simulink model "spring_mass_model_01"  (R2014a)
settings: Solver=FixedStepDiscrete  StartTime=0.0  StopTime=inf  FixedStep=sample_time  RelTol=1e-3
values from neighbouring files (symbols this model uses):
  sample_time = 1/update_freq    (= 0.001)    [init_spring_mass_model_01.m]
undefined symbols (not defined in the file or in its folder): boom_mount_angle, c_energy, contact_threshold, control_start_time, d_y_boom_com_offset, d_y_boom_hip_offset, d_y_mount_to_com, desired_torso_angle, DiscIntNeverNeededParam, dt_thrust, dx_avg_desired, extra_leg_damping, F_thrust, fcut_contact, ff_energy_l, ff_energy_r, g, g_reduced, h_boom, i_limit_lateral, initial_com_height, initial_dt, initial_dx, j_leg, k0_virtual, k_placement, k_sea, kd_flight, kd_lateral, kd_leg_angle, kd_leg_length_secondary, kd_torso, kd_virtual, ki_lateral, kp_flight_max, kp_flight_min, kp_lateral, kp_leg_angle, kp_leg_length_secondary, kp_torso, kp_virtual, l0_virtual, l_boom, l_boom_projected, l_max, l_min, l_retract, l_seg, lambda1, lambda2, lateral_offset, LEG_MTR_MAX_TORQUE, loaded_threshold, m_leg_motor, m_total_real, max_k_virtual, max_leg_angle, max_torque_lateral, min_k_virtual, min_leg_angle ... (+6)
libraries: simulink x22
(part 1 of 2)
settings Model: xpc_rtwmakecfg_data=_xpcethercatlib_  BufferReuse=off  Creator=wmartin  LastModifiedBy=wmartin
settings SolverCC: EnableConcurrentExecution=on
settings DataIOCC: MaxDataPoints=1000000000  SaveFormat=StructureWithTime
settings OptimizationCC: BlockReduction=off  OptimizeBlockIOStorage=off  BufferReuse=off  GlobalBufferReuse=off  ExpressionFolding=off  ExpressionDepthLimit=2147483647  LocalBlockOutputs=off
settings DebuggingCC: UnderspecifiedInitializationDetection=Classic  StateNameClashWarn=warning
settings HardwareCC: ProdIntDivRoundTo=Zero  ProdEndianess=LittleEndian  ProdHWDeviceType=Generic->32-bit x86 compatible
settings RTWCC: SystemTargetFile=slrt.tlc  TemplateMakefile=slrt_default_tmf  Description=Simulink Real-Time  RTWVerbose=off  ProcessScript=slrt_make_rtw_hook  RTWCompilerOptimization=On
settings SimulinkRealTimeCC: GeneratePreprocessorConditionals=Disable all  EnableShiftOperators=on  RL32LogBufSizeModifier=100000000

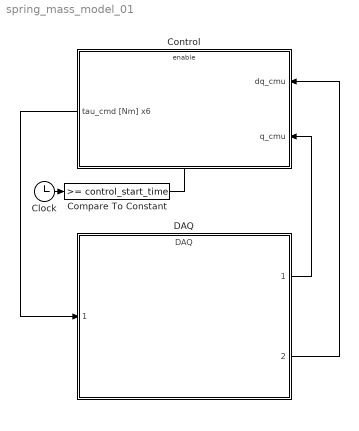
== system spring_mass_model_01 ==
  Clock : Clock
  Compare To Constant : simulink/Logic and Bit Operations/Compare To Constant  relop=>=  const=control_start_time  OutDataTypeStr=boolean
  Control : Subsystem
  DAQ : ModelReference  ModelNameDialog=DAQ  SimulationMode=Normal  ModelReferenceVersion=1.1410  CopyOfModelName=DAQ  DefaultDataLogging=on
  wires:
  DAQ/1 -> Control/2(q_cmu)
  DAQ/2 -> Control/1(dq_cmu)
  Clock/1 -> Compare To Constant/1
  Compare To Constant/1 -> Control/Enable
  Control/1(tau_cmd [Nm] x6) -> DAQ/1

== system spring_mass_model_01/Control ==
  dq_cmu : Inport
  q_cmu : Inport  Port=2
  Enable : EnablePort  StatesWhenEnabling=reset
  Actuator Control : ModelReference  ModelNameDialog=Actuator_Control  SimulationMode=Normal  ModelReferenceVersion=1.5  CopyOfModelName=Actuator_Control  DefaultDataLogging=on
  Behavior Control : Subsystem
  tau_cmd [Nm] x6 : Outport  InitialOutput=[0 0 0 0 0 0]
  wires:
  Behavior Control/1(motor_torque_cmd) -> Actuator Control/1
  dq_cmu/1 -> Actuator Control/3, Behavior Control/1(dq_cmu)
  Actuator Control/1 -> tau_cmd [Nm] x6/1
  q_cmu/1 -> Actuator Control/2, Behavior Control/2(q_cmu)

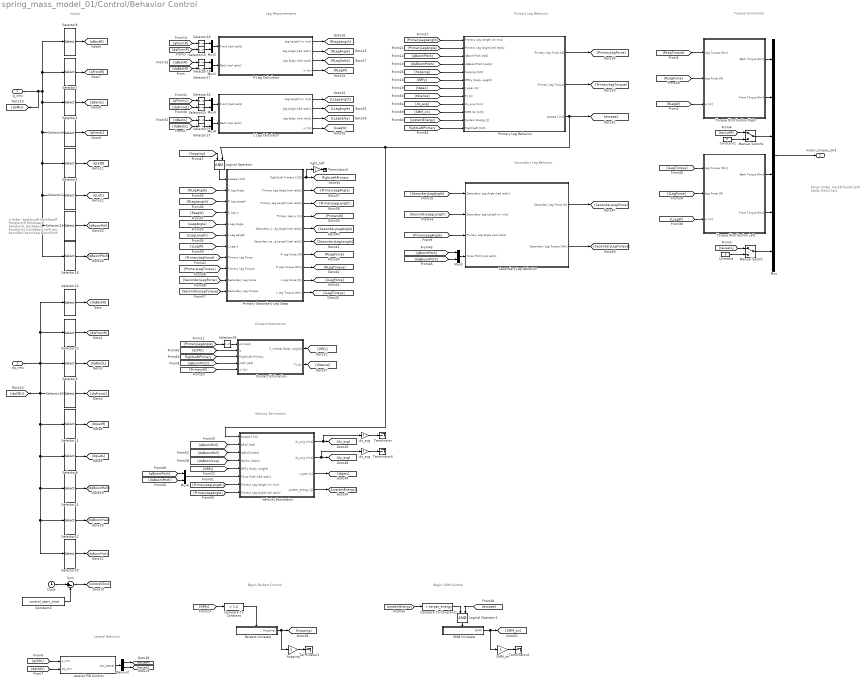
== system spring_mass_model_01/Control/Behavior Control ==
  note: Motor Order:
      |
      | backR
      | frontR
      | latR
      | backL
      | frontL
      | latL
  note: q Order:
      |
      | backJointR
      | backGearR
      | frontJointR
      | frontGearR
      |
      | backJointL
      | backGearL
      | frontJointL
      | frontGearL
      |
      | latR
      | latL
      |
      | boomRoll
      | boomYaw
      | boomPitch
  note: Inputs
  note: Primary Leg Behavior
  note: Secondary Leg Behavior
  note: Torque Commands
  note: Lateral Behavior
  note: Leg Measurements
  note: Contact Estimation
  note: Velocity Estimation
  note: Begin SMM Control
  note: Begin Raibert Control
  dq_cmu : Inport
  q_cmu : Inport  Port=2
  Clock : Clock
  Compare To Constant : simulink/Logic and Bit Operations/Compare To Constant  relop=>  const=1.4  OutDataTypeStr=boolean
  Compare To Constant1 : simulink/Logic and Bit Operations/Compare To Constant  relop=>  const=target_energy  OutDataTypeStr=boolean
  Constant : Constant  Value=0
  Constant1 : Constant  Value=0
  Constant2 : Constant  Value=control_start_time
  Contact Estimation : Subsystem
  Demux2 : Demux  Outputs=2
  L Leg Calculator : Subsystem
  Lateral PID Control : Subsystem
  Logical Operator : Logic  IconShape=distinctive  AllPortsSameDT=off  OutDataTypeStr=boolean
  Logical Operator1 : Logic  IconShape=distinctive  AllPortsSameDT=off  OutDataTypeStr=boolean
  Manual Switch : ManualSwitch
  Manual Switch1 : ManualSwitch
  Mux : Mux  Inputs=6
  Mux{1..6} (6 alike) : Mux  Inputs=2
  Primary Leg Behavior : Subsystem
  Primary Secondary Leg Swap : Subsystem
  R Leg Calculator : Subsystem
  Raibert Initiated : Subsystem
  SMM Initiated : Subsystem
  SMM_on : Gain
  Secondary Leg Behavior : Subsystem
  Selector1 : Selector  InputPortWidth=13  Indices=[10]
  Selector10 : Selector  InputPortWidth=13  Indices=[7 8]
  Selector11 : Selector  InputPortWidth=13  Indices=[9]
  Selector12 : Selector  InputPortWidth=13  Indices=[1 2]
  Selector13 : Selector  InputPortWidth=13  Indices=[3 4]
  Selector{14..17,19,24..27} (9 alike) : Selector  InputPortWidth=2  Indices=[1]
  Selector18 : Selector  InputPortWidth=13  Indices=[13]
  Selector2 : Selector  InputPortWidth=13  Indices=[5 6]
  Selector20 : Selector  InputPortWidth=13  Indices=[13]
  Selector21 : Selector  InputPortWidth=13  Indices=[11]
  Selector22 : Selector  InputPortWidth=13  Indices=[12]
  Selector23 : Selector  InputPortWidth=13  Indices=[11]
  Selector4 : Selector  InputPortWidth=13  Indices=[7 8]
  Selector5 : Selector  InputPortWidth=13  Indices=[9]
  Selector6 : Selector  InputPortWidth=13  Indices=[1 2]
  Selector7 : Selector  InputPortWidth=13  Indices=[3 4]
  Selector8 : Selector  InputPortWidth=13  Indices=[10]
  Selector9 : Selector  InputPortWidth=13  Indices=[5 6]
  Sum : Sum  Inputs=|+-
  Terminator{,1..2,4..5} (5 alike) : Terminator
  Torque Distribution Left : Subsystem
  Torque Distribution Right : Subsystem
  Velocity Estimation : Subsystem
  dx_avg : Gain
  dy_avg : Gain
  hopping : Gain
  right_left : Gain
  motor_torque_cmd : Outport  OutputWhenDisabled=reset  InitialOutput=[0 0 0 0 0 0]
  tag scope: RightLeftPrimary=global
  wires:
  Lateral PID Control/1(tau_lateral) -> Demux2/1
  [dqCMU] -> Lateral PID Control/2(dq_cmu)
  [qCMU] -> Lateral PID Control/1(q_cmu)
  Sum/1 -> [controlClock]
  Selector4/1 -> [qFrontL]
  Selector2/1 -> [qBackL]
  Selector7/1 -> [qFrontR]
  Selector6/1 -> [qBackR]
  Selector1/1 -> [qLatL]
  Selector5/1 -> [qLatR]
  Constant2/1 -> Sum/2
  Clock/1 -> Sum/1
  Constant1/1 -> Manual Switch1/2
  Constant/1 -> Manual Switch/2
  Manual Switch/1 -> Mux/6
  Manual Switch1/1 -> Mux/3
  Mux/1 -> motor_torque_cmd/1
  Selector8/1 -> [dqLatL]
  Selector11/1 -> [dqLatR]
  Selector12/1 -> [dqBackR]
  Selector13/1 -> [dqFrontR]
  Selector9/1 -> [dqBackL]
  Selector10/1 -> [dqFrontL]
  [qBackR] -> Selector16/1
  [dqBackR] -> Selector17/1
  [qFrontR] -> Selector14/1
  [dqFrontR] -> Selector15/1
  Mux2/1 -> R Leg Calculator/1(Front [rad rad/s])
  Mux1/1 -> R Leg Calculator/2(Back [rad rad/s])
  R Leg Calculator/1("Leg Length [m m/s] ") -> [RLegLength]
  R Leg Calculator/2(Leg Angle [rad rad/s]) -> [RLegAngle]
  R Leg Calculator/3(Leg Splay [rad rad/s]) -> [RLegSplay]
  Torque Distribution Right/1(Back Torque [Nm]) -> Mux/1
  Torque Distribution Right/2(Front Torque [Nm]) -> Mux/2
  Demux2/1 -> [tauLatR]
  Demux2/2 -> [tauLatL]
  [tauLatR] -> Manual Switch1/1
  [tauLatL] -> Manual Switch/1
  [RLegW] -> Torque Distribution Right/3(w [m])
  Selector14/1 -> Mux2/1
  Selector15/1 -> Mux2/2
  Selector17/1 -> Mux1/2
  Selector16/1 -> Mux1/1
  [PrimaryW] -> Contact Estimation/5(w [m])
  q_cmu/1 -> Selector6/1, Selector7/1, Selector2/1, Selector4/1, Selector5/1, Selector18/1, Selector23/1, Selector1/1, [qCMU]
  Selector18/1 -> [qBoomPitch]
  [qBoomPitch] -> Contact Estimation/4(pitch [rad])
  [PrimaryLegAngle] -> Selector19/1
  Selector19/1 -> Contact Estimation/1(phi [rad])
  Contact Estimation/1(F_vertical [body weight]) -> [GRFy]
  Selector20/1 -> [dqBoomPitch]
  [RLegForce] -> Torque Distribution Right/2(Leg Force [N])
  [RLegTorque] -> Torque Distribution Right/1(Leg Torque [Nm])
  Selector22/1 -> [dqBoomYaw]
  Contact Estimation/2(Ts [s]) -> [tStance]
  [GRFy] -> Compare To Constant/1
  Raibert Initiated/1(Hopping?) -> hopping/1, [hopping]
  dq_cmu/1 -> Selector20/1, Selector22/1, Selector21/1, Selector8/1, Selector11/1, Selector10/1, [dqCMU], Selector12/1, Selector13/1, Selector9/1
  Selector21/1 -> [dqBoomRoll]
  Selector23/1 -> [qBoomRoll]
  [qBackL] -> Selector26/1
  [dqBackL] -> Selector27/1
  [qFrontL] -> Selector24/1
  [dqFrontL] -> Selector25/1
  Mux5/1 -> L Leg Calculator/1(Front [rad rad/s])
  Mux4/1 -> L Leg Calculator/2(Back [rad rad/s])
  L Leg Calculator/1("Leg Length [m m/s] ") -> [LLegLength]
  L Leg Calculator/2(Leg Angle [rad rad/s]) -> [LLegAngle]
  L Leg Calculator/3(Leg Splay [rad rad/s]) -> [LLegSplay]
  Selector24/1 -> Mux5/1
  Selector25/1 -> Mux5/2
  Selector27/1 -> Mux4/2
  Selector26/1 -> Mux4/1
  R Leg Calculator/4(w [m]) -> [RLegW]
  L Leg Calculator/4(w [m]) -> [LLegW]
  [LLegAngle] -> Primary Secondary Leg Swap/5(L Leg Angle)
  [LLegLength] -> Primary Secondary Leg Swap/6(L Leg Length)
  [LLegW] -> Primary Secondary Leg Swap/7(L Leg w)
  [RLegAngle] -> Primary Secondary Leg Swap/2(R Leg Angle)
  [RLegLength] -> Primary Secondary Leg Swap/3(R Leg Length)
  [RLegW] -> Primary Secondary Leg Swap/4(R Leg w)
  [PrimaryLegForce] -> Primary Secondary Leg Swap/8(Primary Leg Force)
  [PrimaryLegTorque] -> Primary Secondary Leg Swap/9(Primary Leg Torque)
  [SecondaryLegForce] -> Primary Secondary Leg Swap/10(Secondary Leg Force)
  [SecondaryLegTorque] -> Primary Secondary Leg Swap/11(Secondary Leg Torque)
  Primary Secondary Leg Swap/5(Secondary Leg Angle [rad rad/s]) -> [SecondaryLegAngle]
  Primary Secondary Leg Swap/6(Secondary Leg Length [rad rad/s]) -> [SecondaryLegLength]
  Primary Secondary Leg Swap/2(Primary Leg Angle [rad rad/s]) -> [PrimaryLegAngle]
  Primary Secondary Leg Swap/3(Primary Leg Length [rad rad/s]) -> [PrimaryLegLength]
  Primary Secondary Leg Swap/4(Primary Leg w [m]) -> [PrimaryW]
  Primary Secondary Leg Swap/7(R Leg Force [N]) -> [RLegForce]
  Primary Secondary Leg Swap/8(R Leg Torque [Nm]) -> [RLegTorque]
  Primary Secondary Leg Swap/9(L Leg Force [N]) -> [LLegForce]
  Primary Secondary Leg Swap/10(L Leg Torque [Nm]) -> [LLegTorque]
  Primary Leg Behavior/3(escape [1/0]) -> [escape], Velocity Estimation/1(escape [1/0]), Logical Operator/2
  Primary Secondary Leg Swap/1(Right/Left Primary [1/0]) -> right_left/1, [RightLeftPrimary]
  [PrimaryLegLength] -> Primary Leg Behavior/1(Primary Leg Length [m m/s])
  [hopping] -> Primary Leg Behavior/5(hopping [1/0])
  [GRFy] -> Primary Leg Behavior/6(GRFy [body weight])
  [qBoomPitch] -> Primary Leg Behavior/3(qBoomPitch [rad])
  [dqBoomPitch] -> Primary Leg Behavior/4(dqBoomPitch [rad/s])
  [PrimaryLegAngle] -> Primary Leg Behavior/2(Primary Leg Angle [rad rad/s])
  Primary Leg Behavior/1(Primary Leg Force [N]) -> [PrimaryLegForce]
  Primary Leg Behavior/2(Primary Leg Torque) -> [PrimaryLegTorque]
  Velocity Estimation/1(dx_avg [m/s]) -> dx_avg/1, [dx_avg]
  [qBoomRoll] -> Velocity Estimation/2(qRoll [rad])
  [dqBoomYaw] -> Velocity Estimation/4(dqYaw [rad/s])
  dx_avg/1 -> Terminator/1
  hopping/1 -> Terminator1/1
  Torque Distribution Left/1(Back Torque [Nm]) -> Mux/4
  Torque Distribution Left/2(Front Torque [Nm]) -> Mux/5
  [LLegTorque] -> Torque Distribution Left/1(Leg Torque [Nm])
  [LLegForce] -> Torque Distribution Left/2(Leg Force [N])
  [LLegW] -> Torque Distribution Left/3(w [m])
  [qCMU] -> Contact Estimation/2(q)
  [RightLeftPrimary] -> Contact Estimation/3(Right/Left Primary)
  Secondary Leg Behavior/1(Secondary Leg Force [N]) -> [SecondaryLegForce]
  Secondary Leg Behavior/2(Secondary Leg Torque [Nm]) -> [SecondaryLegTorque]
  [PrimaryLegAngle] -> Secondary Leg Behavior/3(Primary Leg Angle [rad rad/s])
  [SecondaryLegAngle] -> Secondary Leg Behavior/1(Secondary Leg Angle [rad rad/s])
  [SecondaryLegLength] -> Secondary Leg Behavior/2(Secondary Leg Length [m m/s])
  [qBoomPitch] -> Mux3/1
  [dqBoomPitch] -> Mux3/2
  Mux3/1 -> Secondary Leg Behavior/4(Torso Pitch [rad rad/s])
  right_left/1 -> Terminator2/1
  [hopping] -> Logical Operator/1
  Logical Operator/1 -> Primary Secondary Leg Swap/1(escape [1/0])
  Compare To Constant/1 -> Raibert Initiated/Enable
  Velocity Estimation/2(dy_avg [m/s]) -> dy_avg/1, [dy_avg]
  [tApex] -> Primary Leg Behavior/7(t_apex [s])
  Velocity Estimation/3(t_apex [s]) -> [tApex]
  [GRFy] -> Velocity Estimation/5(GRFy [body weight])
  Mux6/1 -> Velocity Estimation/6(Torso Pitch [rad rad/s])
  [qBoomPitch] -> Mux6/1
  [dqBoomPitch] -> Mux6/2
  [PrimaryLegAngle] -> Velocity Estimation/8(Primary Leg Angle [rad rad/s])
  [PrimaryLegLength] -> Velocity Estimation/7(Primary Leg Length [m m/s])
  dy_avg/1 -> Terminator5/1
  [dqBoomRoll] -> Velocity Estimation/3(dqRoll [rad/s])
  [dx_avg] -> Primary Leg Behavior/9(dx_avg [m/s])
  [tStance] -> Primary Leg Behavior/8(Ts [s])
  Velocity Estimation/4(system_energy [J]) -> [systemEnergy]
  [systemEnergy] -> Compare To Constant1/1
  SMM Initiated/1(SMM?) -> [SMM_on], SMM_on/1
  SMM_on/1 -> Terminator4/1
  Compare To Constant1/1 -> Logical Operator1/1
  [SMM_on] -> Primary Leg Behavior/10(SMM On [1/0])
  [systemEnergy] -> Primary Leg Behavior/11(System Energy [J])
  Logical Operator1/1 -> SMM Initiated/Enable
  [escape] -> Logical Operator1/2
  [RightLeftPrimary] -> Primary Leg Behavior/12(Right/Left [1/0])

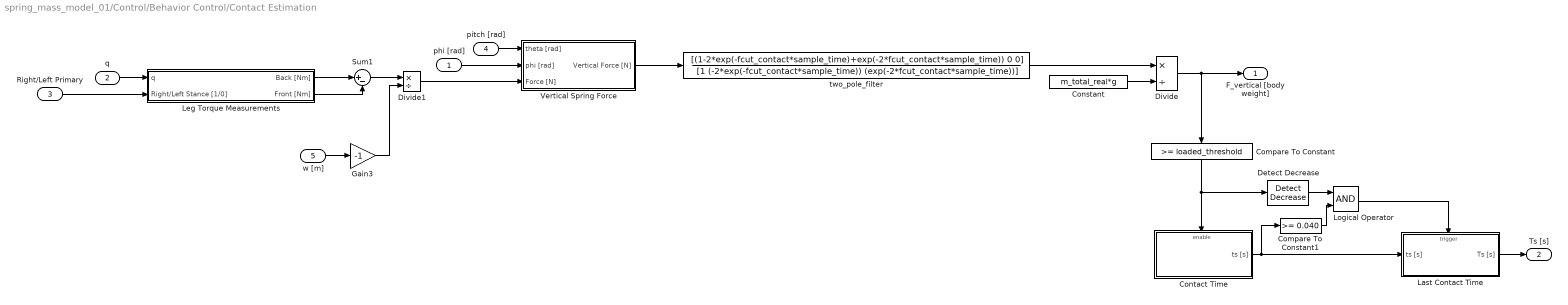
== system spring_mass_model_01/Control/Behavior Control/Contact Estimation ==
  phi [rad] : Inport
  q : Inport  Port=2
  Right/Left Primary : Inport  Port=3
  pitch [rad] : Inport  Port=4
  w [m] : Inport  Port=5
  Compare To Constant : simulink/Logic and Bit Operations/Compare To Constant  relop=>=  const=loaded_threshold  OutDataTypeStr=boolean
  Compare To Constant1 : simulink/Logic and Bit Operations/Compare To Constant  relop=>=  const=0.040  OutDataTypeStr=boolean
  Constant : Constant  Value=m_total_real*g
  Contact Time : Subsystem
  Detect Decrease : simulink/Logic and Bit Operations/Detect Decrease  vinit=0.0  InputProcessing=Inherited  OutDataTypeStr=boolean
  Divide : Product  Inputs=*/
  Divide1 : Product  Inputs=*/
  Gain3 : Gain  Gain=-1
  Last Contact Time : Subsystem
  Leg Torque Measurements : Subsystem
  Logical Operator : Logic  AllPortsSameDT=off  OutDataTypeStr=boolean
  Sum1 : Sum  Inputs=|+-
  Vertical Spring Force : Subsystem
  two_pole_filter : DiscreteTransferFcn  Numerator=[(1-2*exp(-fcut_contact*sample_time)+exp(-2*fcut_contact*sample_time)) 0 0]  Denominator=[1 (-2*exp(-fcut_contact*sample_time)) (exp(-2*fcut_contact*sample_time))]  SampleTime=sample_time
  F_vertical [body weight] : Outport
  Ts [s] : Outport  Port=2
  wires:
  Vertical Spring Force/1(Vertical Force [N]) -> two_pole_filter/1
  Constant/1 -> Divide/2
  two_pole_filter/1 -> Divide/1
  q/1 -> Leg Torque Measurements/1(q)
  Leg Torque Measurements/1(Back [Nm]) -> Sum1/1
  Leg Torque Measurements/2(Front [Nm]) -> Sum1/2
  Sum1/1 -> Divide1/1
  Divide1/1 -> Vertical Spring Force/3(Force [N])
  pitch [rad]/1 -> Vertical Spring Force/1(theta [rad])
  w [m]/1 -> Gain3/1
  Gain3/1 -> Divide1/2
  phi [rad]/1 -> Vertical Spring Force/2(phi [rad])
  Last Contact Time/1(Ts [s]) -> Ts [s]/1
  Contact Time/1(ts [s]) -> Last Contact Time/1(ts [s]), Compare To Constant1/1
  Compare To Constant/1 -> Detect Decrease/1, Contact Time/Enable
  Divide/1 -> F_vertical [body weight]/1, Compare To Constant/1
  Logical Operator/1 -> Last Contact Time/Trigger
  Detect Decrease/1 -> Logical Operator/1
  Compare To Constant1/1 -> Logical Operator/2
  Right/Left Primary/1 -> Leg Torque Measurements/2(Right/Left Stance [1/0])

== system spring_mass_model_01/Control/Behavior Control/L Leg Calculator ==
  Front [rad rad/s] : Inport
  Back [rad rad/s] : Inport  Port=2
  Demux1 : Demux  Outputs=2
  Gain1 : Gain  Gain=2*l_seg
  Gain2 : Gain  Gain=l_seg
  Gain3 : Gain  Gain=-1
  Gain4 : Gain  Gain=0.5
  Gain5 : Gain  Gain=0.5
  Gain6 : Gain  Gain=2
  Mux1 : Mux  Inputs=2
  Product : Product  RndMeth=Zero
  Sum4 : Sum  Inputs=+|+
  Sum5 : Sum  Inputs=+|-
  Trigonometric Function : Trigonometry  Operator=cos
  Trigonometric Function1 : Trigonometry
  "Leg Length [m m/s] " : Outport
  Leg Angle [rad rad/s] : Outport  Port=2
  Leg Splay [rad rad/s] : Outport  Port=3
  w [m] : Outport  Port=4
  wires:
  Gain5/1 -> Leg Angle [rad rad/s]/1
  Sum4/1 -> Gain5/1
  Mux1/1 -> "Leg Length [m m/s] "/1
  Sum5/1 -> Demux1/1, Leg Splay [rad rad/s]/1
  Gain2/1 -> Gain6/1, Product/1
  Demux1/1 -> Gain4/1
  Gain3/1 -> Product/2
  Demux1/2 -> Gain3/1
  Back [rad rad/s]/1 -> Sum5/1, Sum4/1
  Front [rad rad/s]/1 -> Sum4/2, Sum5/2
  Product/1 -> Mux1/2
  Trigonometric Function1/1 -> Gain2/1
  Gain1/1 -> Mux1/1
  Trigonometric Function/1 -> Gain1/1
  Gain4/1 -> Trigonometric Function/1, Trigonometric Function1/1
  Gain6/1 -> w [m]/1

== system spring_mass_model_01/Control/Behavior Control/Lateral PID Control ==
  note: FB Linearization
  q_cmu : Inport
  dq_cmu : Inport  Port=2
  -mgd : Gain  Gain=m_leg_motor*g*lateral_offset
  90deg : Constant  Value=pi/2
  Gain : Gain  Gain=-1
  Lateral Hip PID : Subsystem
  Motor Saturation : Saturate  UpperLimit=max_torque_lateral  LowerLimit=-max_torque_lateral
      settings: AttributesFormatString=Top: %<UpperLimit>\nBottom: %<LowerLimit>
  Mux : Mux  Inputs=2
  Sum1 : Sum  Inputs=|+-
  Sum2 : Sum  Inputs=-+|
  Sum3 : Sum  Inputs=++|
  Sum4 : Sum  Inputs=++|
  desired_velocity : Constant  Value=0
  lateral_sine : Gain  Commented=on  Gain=pi/180
  lateral_wave : Sin  Commented=on  Amplitude=5  Frequency=2*pi*(1/2)  SampleTime=0
  select_dqLateral : Selector  InputPortWidth=13  Indices=[9 10]
  select_qLateral : Selector  InputPortWidth=13  Indices=[9 10]
  sin : Trigonometry
  spherical_correction_angle : Subsystem
  tau_lateral : Outport
  wires:
  lateral_wave/1 -> lateral_sine/1
  Lateral Hip PID/1(out) -> Sum4/2
  Sum2/1 -> Lateral Hip PID/1(position_error)
  q_cmu/1 -> spherical_correction_angle/1(q_cmu), select_qLateral/1
  select_dqLateral/1 -> Sum1/2
  dq_cmu/1 -> select_dqLateral/1
  Sum4/1 -> Motor Saturation/1
  desired_velocity/1 -> Sum1/1
  Sum1/1 -> Lateral Hip PID/2(velocity_error)
  Gain/1 -> Mux/2
  Mux/1 -> Sum2/2
  select_qLateral/1 -> Sum3/2, Sum2/1  "qLateral"
  Motor Saturation/1 -> tau_lateral/1
  spherical_correction_angle/1(lateral_correction [rad]) -> Mux/1, Gain/1
  -mgd/1 -> Sum4/1
  Sum3/1 -> sin/1
  90deg/1 -> Sum3/1
  sin/1 -> -mgd/1

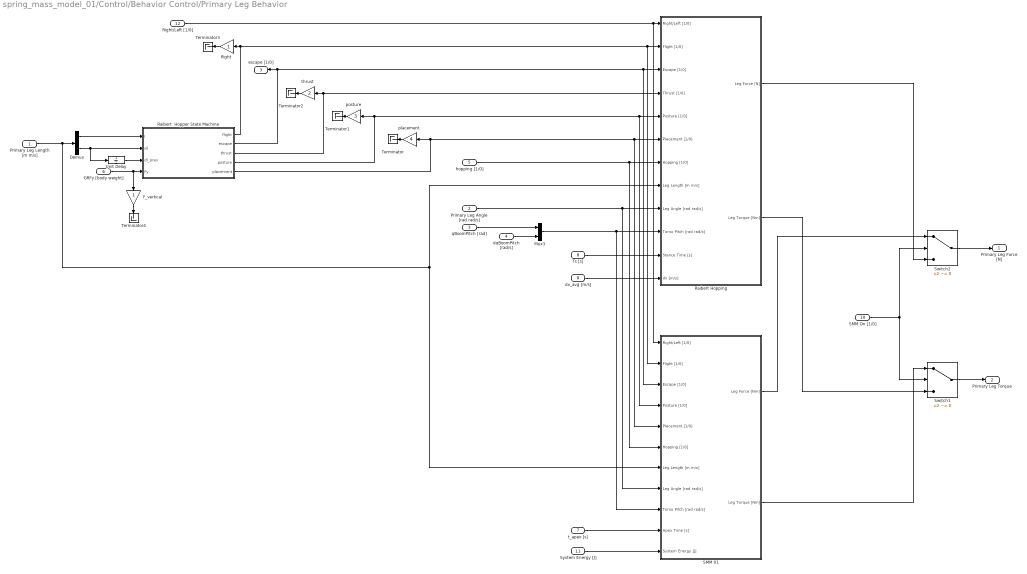
== system spring_mass_model_01/Control/Behavior Control/Primary Leg Behavior ==
  Primary Leg Length [m m/s] : Inport
  Primary Leg Angle [rad rad/s] : Inport  Port=2
  qBoomPitch [rad] : Inport  Port=3
  dqBoomPitch [rad/s] : Inport  Port=4
  hopping [1/0] : Inport  Port=5
  GRFy [body weight] : Inport  Port=6
  t_apex [s] : Inport  Port=7
  Ts [s] : Inport  Port=8
  dx_avg [m/s] : Inport  Port=9
  SMM On [1/0] : Inport  Port=10
  System Energy [J] : Inport  Port=11
  Right/Left [1/0] : Inport  Port=12
  Demux : Demux  Outputs=2
  F_vertical : Gain
  Mux3 : Mux  Inputs=2
  Raibert  Hopper State Machine : State Transition Table  TreatAsAtomicUnit=on
  Raibert Hopping : Subsystem
  SMM 01 : Subsystem
  Switch1 : Switch  Criteria=u2 ~= 0
  Switch2 : Switch  Criteria=u2 ~= 0
  Terminator{,1..4} (5 alike) : Terminator
  Unit Delay : UnitDelay  SampleTime=-1
  flight : Gain
  placement : Gain  Gain=4
  posture : Gain  Gain=3
  thrust : Gain  Gain=2
  Primary Leg Force [N] : Outport
  Primary Leg Torque : Outport  Port=2
  escape [1/0] : Outport  Port=3
  wires:
  Raibert  Hopper State Machine/4(posture) -> SMM 01/4(Posture [1/0]), Raibert Hopping/5(Posture [1/0]), posture/1
  Mux3/1 -> SMM 01/9(Torso Pitch [rad rad/s]), Raibert Hopping/10(Torso Pitch [rad rad/s])
  qBoomPitch [rad]/1 -> Mux3/1
  dqBoomPitch [rad/s]/1 -> Mux3/2
  Unit Delay/1 -> Raibert  Hopper State Machine/3(dl_prev)
  GRFy [body weight]/1 -> F_vertical/1, Raibert  Hopper State Machine/4(Fy)
  Demux/2 -> Unit Delay/1, Raibert  Hopper State Machine/2(dl)
  Raibert  Hopper State Machine/3(thrust) -> thrust/1, Raibert Hopping/4(Thrust [1/0])
  Raibert  Hopper State Machine/1(flight) -> flight/1, SMM 01/2(Flight [1/0]), Raibert Hopping/2(Flight [1/0])
  Raibert  Hopper State Machine/2(escape) -> SMM 01/3(Escape [1/0]), Raibert Hopping/3(Escape [1/0]), escape [1/0]/1
  Raibert  Hopper State Machine/5(placement) -> Raibert Hopping/6(Placement [1/0]), SMM 01/5(Placement [1/0]), placement/1
  placement/1 -> Terminator/1
  posture/1 -> Terminator1/1
  thrust/1 -> Terminator2/1
  Primary Leg Length [m m/s]/1 -> SMM 01/7(Leg Length [m m/s]), Raibert Hopping/8(Leg Length [m m/s]), Demux/1
  F_vertical/1 -> Terminator4/1
  flight/1 -> Terminator3/1
  Demux/1 -> Raibert  Hopper State Machine/1(l)
  hopping [1/0]/1 -> SMM 01/6(Hopping [1/0]), Raibert Hopping/7(Hopping [1/0])
  SMM On [1/0]/1 -> Switch1/2, Switch2/2
  Ts [s]/1 -> Raibert Hopping/11(Stance Time [s])
  dx_avg [m/s]/1 -> Raibert Hopping/12(dx [m/s])
  Raibert Hopping/1(Leg Force [N]) -> Switch2/3
  Raibert Hopping/2(Leg Torque [Nm]) -> Switch1/3
  Switch2/1 -> Primary Leg Force [N]/1
  Switch1/1 -> Primary Leg Torque/1
  t_apex [s]/1 -> SMM 01/10(Apex Time [s])
  System Energy [J]/1 -> SMM 01/11(System Energy [J])
  Primary Leg Angle [rad rad/s]/1 -> SMM 01/8(Leg Angle [rad rad/s]), Raibert Hopping/9(Leg Angle [rad rad/s])
  SMM 01/1(Leg Force [Nm]) -> Switch2/1
  SMM 01/2(Leg Torque [Nm]) -> Switch1/1
  Right/Left [1/0]/1 -> SMM 01/1(Right/Left [1/0]), Raibert Hopping/1(Right/Left [1/0])

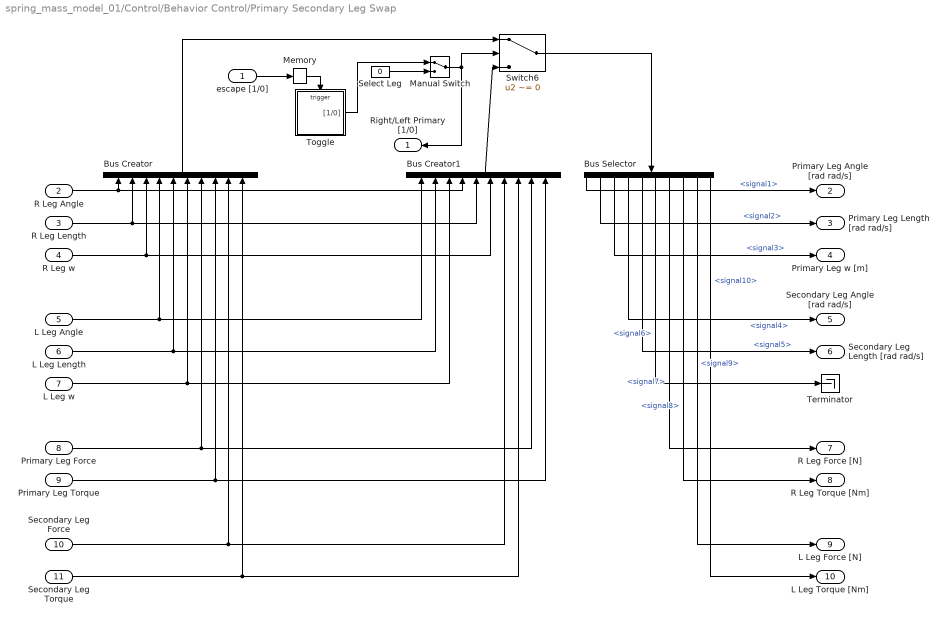
== system spring_mass_model_01/Control/Behavior Control/Primary Secondary Leg Swap ==
  escape [1/0] : Inport
  R Leg Angle : Inport  Port=2
  R Leg Length : Inport  Port=3
  R Leg w : Inport  Port=4
  L Leg Angle : Inport  Port=5
  L Leg Length : Inport  Port=6
  L Leg w : Inport  Port=7
  Primary Leg Force : Inport  Port=8
  Primary Leg Torque : Inport  Port=9
  Secondary Leg Force : Inport  Port=10
  Secondary Leg Torque : Inport  Port=11
  Bus Creator : BusCreator  Inputs=10
  Bus Creator1 : BusCreator  Inputs=10
  Bus Selector : BusSelector  OutputSignals=signal1,signal2,signal3,signal4,signal5,signal6,signal7,signal8,signal9,signal10
  Manual Switch : ManualSwitch
  Memory : Memory  InheritSampleTime=on
  Select Leg : Constant  Value=0  OutDataTypeStr=boolean
  Switch6 : Switch  Criteria=u2 ~= 0  ZeroCross=off
  Terminator : Terminator
  Toggle : Subsystem
  Right/Left Primary [1/0] : Outport
  Primary Leg Angle [rad rad/s] : Outport  Port=2
  Primary Leg Length [rad rad/s] : Outport  Port=3
  Primary Leg w [m] : Outport  Port=4
  Secondary Leg Angle [rad rad/s] : Outport  Port=5
  Secondary Leg Length [rad rad/s] : Outport  Port=6
  R Leg Force [N] : Outport  Port=7
  R Leg Torque [Nm] : Outport  Port=8
  L Leg Force [N] : Outport  Port=9
  L Leg Torque [Nm] : Outport  Port=10
  wires:
  Memory/1 -> Toggle/Trigger
  Toggle/1("[1/0]") -> Manual Switch/1
  Manual Switch/1 -> Right/Left Primary [1/0]/1, Switch6/2
  Select Leg/1 -> Manual Switch/2
  Bus Selector/10 -> L Leg Torque [Nm]/1  "<signal10>"
  Bus Selector/9 -> L Leg Force [N]/1  "<signal9>"
  Bus Selector/8 -> R Leg Torque [Nm]/1  "<signal8>"
  Bus Selector/7 -> R Leg Force [N]/1  "<signal7>"
  Bus Selector/6 -> Terminator/1  "<signal6>"
  Bus Selector/5 -> Secondary Leg Length [rad rad/s]/1  "<signal5>"
  Bus Selector/4 -> Secondary Leg Angle [rad rad/s]/1  "<signal4>"
  Bus Selector/3 -> Primary Leg w [m]/1  "<signal3>"
  Bus Selector/2 -> Primary Leg Length [rad rad/s]/1  "<signal2>"
  Bus Selector/1 -> Primary Leg Angle [rad rad/s]/1  "<signal1>"
  L Leg Angle/1 -> Bus Creator1/1, Bus Creator/4
  L Leg Length/1 -> Bus Creator1/2, Bus Creator/5
  Primary Leg Force/1 -> Bus Creator/7, Bus Creator1/9
  R Leg w/1 -> Bus Creator/3, Bus Creator1/6
  R Leg Angle/1 -> Bus Creator/1, Bus Creator1/4
  L Leg w/1 -> Bus Creator1/3, Bus Creator/6
  R Leg Length/1 -> Bus Creator/2, Bus Creator1/5
  escape [1/0]/1 -> Memory/1
  Secondary Leg Force/1 -> Bus Creator/9, Bus Creator1/7
  Secondary Leg Torque/1 -> Bus Creator/10, Bus Creator1/8
  Primary Leg Torque/1 -> Bus Creator/8, Bus Creator1/10
  Bus Creator/1 -> Switch6/1
  Bus Creator1/1 -> Switch6/3
  Switch6/1 -> Bus Selector/1

== system spring_mass_model_01/Control/Behavior Control/R Leg Calculator ==
  Front [rad rad/s] : Inport
  Back [rad rad/s] : Inport  Port=2
  Demux1 : Demux  Outputs=2
  Gain1 : Gain  Gain=2*l_seg
  Gain2 : Gain  Gain=l_seg
  Gain3 : Gain  Gain=-1
  Gain4 : Gain  Gain=0.5
  Gain5 : Gain  Gain=0.5
  Gain6 : Gain  Gain=2
  Mux1 : Mux  Inputs=2
  Product : Product  RndMeth=Zero
  Sum4 : Sum  Inputs=+|+
  Sum5 : Sum  Inputs=+|-
  Trigonometric Function : Trigonometry  Operator=cos
  Trigonometric Function1 : Trigonometry
  "Leg Length [m m/s] " : Outport
  Leg Angle [rad rad/s] : Outport  Port=2
  Leg Splay [rad rad/s] : Outport  Port=3
  w [m] : Outport  Port=4
  wires:
  Gain6/1 -> w [m]/1
  Gain4/1 -> Trigonometric Function1/1, Trigonometric Function/1
  Trigonometric Function/1 -> Gain1/1
  Gain1/1 -> Mux1/1
  Trigonometric Function1/1 -> Gain2/1
  Product/1 -> Mux1/2
  Front [rad rad/s]/1 -> Sum5/2, Sum4/2
  Back [rad rad/s]/1 -> Sum4/1, Sum5/1
  Demux1/2 -> Gain3/1
  Gain3/1 -> Product/2
  Demux1/1 -> Gain4/1
  Gain2/1 -> Product/1, Gain6/1
  Sum5/1 -> Leg Splay [rad rad/s]/1, Demux1/1
  Mux1/1 -> "Leg Length [m m/s] "/1
  Sum4/1 -> Gain5/1
  Gain5/1 -> Leg Angle [rad rad/s]/1

== system spring_mass_model_01/Control/Behavior Control/Raibert Initiated ==
  Enable : EnablePort  StatesWhenEnabling=reset
  Constant : Constant
  Hopping? : Outport  InitialOutput=[0]
  wires:
  Constant/1 -> Hopping?/1

== system spring_mass_model_01/Control/Behavior Control/SMM Initiated ==
  Enable : EnablePort  StatesWhenEnabling=reset
  Constant : Constant
  SMM? : Outport  InitialOutput=[0]
  wires:
  Constant/1 -> SMM?/1

== system spring_mass_model_01/Control/Behavior Control/Secondary Leg Behavior ==
  Secondary Leg Angle [rad rad/s] : Inport
  Secondary Leg Length [m m/s] : Inport  Port=2
  Primary Leg Angle [rad rad/s] : Inport  Port=3
  Torso Pitch [rad rad/s] : Inport  Port=4
  Constant12 : Constant  Value=0.75
  Constant9 : Constant  Value=0
  Demux5 : Demux  Outputs=2
  Fcn2 : Fcn  Expr=2*pi-u(1)
  Leg Angle PD : Subsystem
  Leg Length PD : Subsystem
  Sum1 : Sum  Inputs=|++
  Sum2 : Sum  Inputs=|++
  k_virtual6 : Gain  Gain=-1
  Secondary Leg Force [N] : Outport
  Secondary Leg Torque [Nm] : Outport  Port=2
  wires:
  Leg Angle PD/1(Commanded Leg Torque [Nm]) -> Secondary Leg Torque [Nm]/1
  Demux5/2 -> k_virtual6/1
  Demux5/1 -> Fcn2/1
  Sum1/1 -> Demux5/1
  k_virtual6/1 -> Leg Angle PD/2(Desired Velocity)
  Fcn2/1 -> Leg Angle PD/1(Desired Angle)
  Sum2/1 -> Leg Angle PD/3(Leg Angle [rad rad/s])
  Torso Pitch [rad rad/s]/1 -> Sum2/2, Sum1/2
  Secondary Leg Angle [rad rad/s]/1 -> Sum2/1
  Leg Length PD/1(Commanded Force [N]) -> Secondary Leg Force [N]/1
  Secondary Leg Length [m m/s]/1 -> Leg Length PD/3(Leg Length [m m/s])
  Constant12/1 -> Leg Length PD/1(Desired Length)
  Constant9/1 -> Leg Length PD/2(Desired Velocity)
  Primary Leg Angle [rad rad/s]/1 -> Sum1/1

== system spring_mass_model_01/Control/Behavior Control/Torque Distribution Left ==
  Leg Torque [Nm] : Inport
  Leg Force [N] : Inport  Port=2
  w [m] : Inport  Port=3
  Gain : Gain  Gain=0.5
  Gain1 : Gain  Gain=0.5
  Motor Torque Saturation Optimization : MATLAB Function  TreatAsAtomicUnit=on
  Product : Product  RndMeth=Zero
  Sum : Sum  Inputs=|++
  Sum1 : Sum  Inputs=+-|
  Back Torque [Nm] : Outport
  Front Torque [Nm] : Outport  Port=2
  wires:
  Sum1/1 -> Back Torque [Nm]/1
  Leg Torque [Nm]/1 -> Gain/1
  Sum/1 -> Front Torque [Nm]/1
  Motor Torque Saturation Optimization/1(t1) -> Sum/1, Sum1/1
  w [m]/1 -> Product/2
  Motor Torque Saturation Optimization/2(t2) -> Sum1/2, Sum/2
  Leg Force [N]/1 -> Product/1
  Product/1 -> Gain1/1
  Gain1/1 -> Motor Torque Saturation Optimization/2(x2s)
  Gain/1 -> Motor Torque Saturation Optimization/1(x1s)

== system spring_mass_model_01/Control/Behavior Control/Torque Distribution Right ==
  Leg Torque [Nm] : Inport
  Leg Force [N] : Inport  Port=2
  w [m] : Inport  Port=3
  Gain : Gain  Gain=0.5
  Gain1 : Gain  Gain=0.5
  Motor Torque Saturation Optimization : MATLAB Function  TreatAsAtomicUnit=on
  Product : Product  RndMeth=Zero
  Sum : Sum  Inputs=|++
  Sum1 : Sum  Inputs=+-|
  Back Torque [Nm] : Outport
  Front Torque [Nm] : Outport  Port=2
  wires:
  Gain/1 -> Motor Torque Saturation Optimization/1(x1s)
  Gain1/1 -> Motor Torque Saturation Optimization/2(x2s)
  Product/1 -> Gain1/1
  Leg Force [N]/1 -> Product/1
  Motor Torque Saturation Optimization/2(t2) -> Sum/2, Sum1/2
  w [m]/1 -> Product/2
  Motor Torque Saturation Optimization/1(t1) -> Sum1/1, Sum/1
  Sum/1 -> Front Torque [Nm]/1
  Leg Torque [Nm]/1 -> Gain/1
  Sum1/1 -> Back Torque [Nm]/1

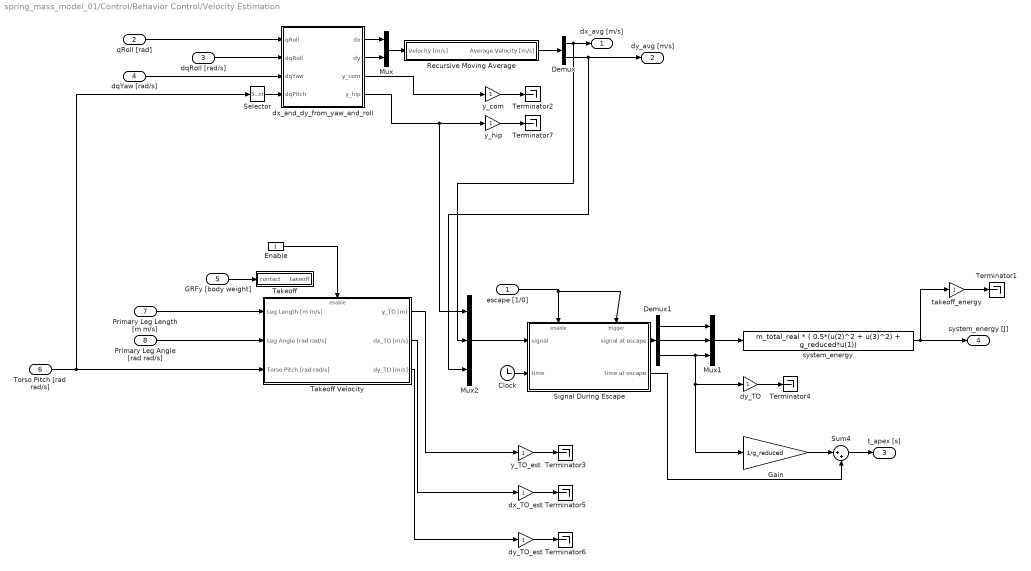
== system spring_mass_model_01/Control/Behavior Control/Velocity Estimation ==
  escape [1/0] : Inport
  qRoll [rad] : Inport  Port=2
  dqRoll [rad/s] : Inport  Port=3
  dqYaw [rad/s] : Inport  Port=4
  GRFy [body weight] : Inport  Port=5
  Torso Pitch [rad rad/s] : Inport  Port=6
  Primary Leg Length [m m/s] : Inport  Port=7
  Primary Leg Angle [rad rad/s] : Inport  Port=8
  Clock : Clock
  Demux : Demux  Outputs=2
  Demux1 : Demux  Outputs=3
  Enable : Constant  OutDataTypeStr=boolean
  Gain : Gain  Gain=1/g_reduced
  Mux : Mux  Inputs=2
  Mux1 : Mux  Inputs=3
  Mux2 : Mux  Inputs=3
  Recursive Moving Average : Subsystem
  Selector : Selector  InputPortWidth=2  Indices=[2]
  Signal During Escape : Subsystem
  Sum4 : Sum  Inputs=|++
  Takeoff : Subsystem
  Takeoff Velocity : Subsystem
  Terminator{1..7} (7 alike) : Terminator
  dx_TO_est : Gain
  dx_and_dy_from_yaw_and_roll : MATLAB Function  TreatAsAtomicUnit=on
  dy_TO : Gain
  dy_TO_est : Gain
  system_energy : Fcn  Expr=m_total_real * ( 0.5*(u(2)^2 + u(3)^2) + g_reduced*u(1))
  takeoff_energy : Gain
  y_TO_est : Gain
  y_com : Gain
  y_hip : Gain
  dx_avg [m/s] : Outport
  dy_avg [m/s] : Outport  Port=2
  t_apex [s] : Outport  Port=3
  system_energy [J] : Outport  Port=4
  wires:
  Recursive Moving Average/1(Average Velocity [m/s]) -> Demux/1
  dx_and_dy_from_yaw_and_roll/1(dx) -> Mux/1
  dqYaw [rad/s]/1 -> dx_and_dy_from_yaw_and_roll/3(dqYaw)
  Selector/1 -> dx_and_dy_from_yaw_and_roll/4(dqPitch)
  GRFy [body weight]/1 -> Takeoff/1(contact)
  dx_and_dy_from_yaw_and_roll/2(dy) -> Mux/2
  Mux/1 -> Recursive Moving Average/1(Velocity [m/s])
  Demux/1 -> Mux2/2, dx_avg [m/s]/1
  Demux/2 -> Mux2/3, dy_avg [m/s]/1
  Sum4/1 -> t_apex [s]/1
  Primary Leg Length [m m/s]/1 -> Takeoff Velocity/1(Leg Length [m m/s])
  Primary Leg Angle [rad rad/s]/1 -> Takeoff Velocity/2(Leg Angle [rad rad/s])
  Torso Pitch [rad rad/s]/1 -> Selector/1, Takeoff Velocity/3(Torso Pitch [rad rad/s])
  Demux1/2 -> Mux1/2
  Demux1/1 -> Mux1/1
  Mux1/1 -> system_energy/1
  dy_TO/1 -> Terminator4/1
  takeoff_energy/1 -> Terminator1/1
  dqRoll [rad/s]/1 -> dx_and_dy_from_yaw_and_roll/2(dqRoll)
  escape [1/0]/1 -> Signal During Escape/Trigger, Signal During Escape/Enable
  Mux2/1 -> Signal During Escape/1(signal)
  Signal During Escape/1(signal at escape) -> Demux1/1
  qRoll [rad]/1 -> dx_and_dy_from_yaw_and_roll/1(qRoll)
  dx_and_dy_from_yaw_and_roll/3(y_com) -> y_com/1
  Signal During Escape/2(time at escape) -> Sum4/2
  Gain/1 -> Sum4/1
  Demux1/3 -> Gain/1, dy_TO/1, Mux1/3
  Clock/1 -> Signal During Escape/2(time)
  system_energy/1 -> system_energy [J]/1, takeoff_energy/1
  y_com/1 -> Terminator2/1
  Takeoff Velocity/1(y_TO [m]) -> y_TO_est/1
  y_TO_est/1 -> Terminator3/1
  dx_TO_est/1 -> Terminator5/1
  Takeoff Velocity/2(dx_TO [m/s]) -> dx_TO_est/1
  dy_TO_est/1 -> Terminator6/1
  Takeoff Velocity/3(dy_TO [m/s]) -> dy_TO_est/1
  y_hip/1 -> Terminator7/1
  dx_and_dy_from_yaw_and_roll/4(y_hip) -> Mux2/1, y_hip/1
  Enable/1 -> Takeoff Velocity/Enable

== system spring_mass_model_01/Control/Behavior Control/Contact Estimation/Contact Time ==
  Enable : EnablePort  StatesWhenEnabling=reset  ShowOutputPort=on
  Constant : Constant
  Discrete-Time Integrator : DiscreteIntegrator  IntegratorMethod=Accumulation: Forward Euler  gainval=sample_time  ExternalReset=rising  SampleTime=sample_time  ICPrevOutput=DiscIntNeverNeededParam  ICPrevScaledInput=DiscIntNeverNeededParam
  ts [s] : Outport  InitialOutput=[0]
  wires:
  Constant/1 -> Discrete-Time Integrator/1
  Enable/1 -> Discrete-Time Integrator/2
  Discrete-Time Integrator/1 -> ts [s]/1

== system spring_mass_model_01/Control/Behavior Control/Contact Estimation/Last Contact Time ==
  ts [s] : Inport
  Trigger : TriggerPort  TriggerType=falling  PortDimensions=1
  Ts [s] : Outport  InitialOutput=[initial_dt]
  wires:
  ts [s]/1 -> Ts [s]/1

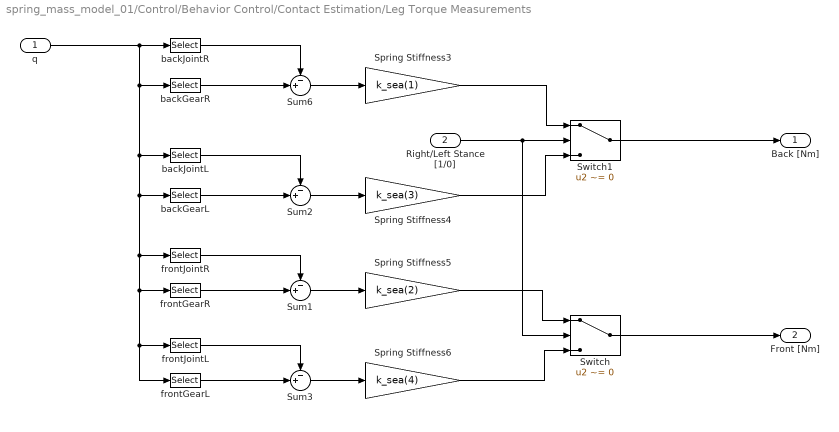
== system spring_mass_model_01/Control/Behavior Control/Contact Estimation/Leg Torque Measurements ==
  q : Inport
  Right/Left Stance [1/0] : Inport  Port=2
  Spring Stiffness3 : Gain  Gain=k_sea(1)
  Spring Stiffness4 : Gain  Gain=k_sea(3)
  Spring Stiffness5 : Gain  Gain=k_sea(2)
  Spring Stiffness6 : Gain  Gain=k_sea(4)
  Sum{1..3,6} (4 alike) : Sum  Inputs=-+|
  Switch : Switch  Criteria=u2 ~= 0
  Switch1 : Switch  Criteria=u2 ~= 0
  backGearL : Selector  InputPortWidth=13  Indices=[6]
  backGearR : Selector  InputPortWidth=13  Indices=[2]
  backJointL : Selector  InputPortWidth=13  Indices=[5]
  backJointR : Selector  InputPortWidth=13  Indices=[1]
  frontGearL : Selector  InputPortWidth=13  Indices=[8]
  frontGearR : Selector  InputPortWidth=13  Indices=[4]
  frontJointL : Selector  InputPortWidth=13  Indices=[7]
  frontJointR : Selector  InputPortWidth=13  Indices=[3]
  Back [Nm] : Outport
  Front [Nm] : Outport  Port=2
  wires:
  Spring Stiffness6/1 -> Switch/3
  Spring Stiffness5/1 -> Switch/1
  Spring Stiffness4/1 -> Switch1/3
  Spring Stiffness3/1 -> Switch1/1
  q/1 -> backJointR/1, frontGearL/1, frontJointL/1, frontGearR/1, frontJointR/1, backGearL/1, backJointL/1, backGearR/1
  backGearR/1 -> Sum6/2
  frontJointR/1 -> Sum1/1
  frontGearR/1 -> Sum1/2
  backJointR/1 -> Sum6/1
  Switch/1 -> Front [Nm]/1
  Sum1/1 -> Spring Stiffness5/1
  Sum6/1 -> Spring Stiffness3/1
  backGearL/1 -> Sum2/2
  frontJointL/1 -> Sum3/1
  frontGearL/1 -> Sum3/2
  backJointL/1 -> Sum2/1
  Switch1/1 -> Back [Nm]/1
  Sum2/1 -> Spring Stiffness4/1
  Sum3/1 -> Spring Stiffness6/1
  Right/Left Stance [1/0]/1 -> Switch/2, Switch1/2

== system spring_mass_model_01/Control/Behavior Control/Contact Estimation/Vertical Spring Force ==
  theta [rad] : Inport
  phi [rad] : Inport  Port=2
  Force [N] : Inport  Port=3
  Gain : Gain  Gain=-1
  Product : Product
  Sum : Sum  Inputs=++|
  Trigonometric Function : Trigonometry  Operator=cos
  Vertical Force [N] : Outport
  wires:
  Force [N]/1 -> Product/1
  phi [rad]/1 -> Sum/2
  theta [rad]/1 -> Sum/1
  Trigonometric Function/1 -> Product/2
  Product/1 -> Gain/1
  Sum/1 -> Trigonometric Function/1
  Gain/1 -> Vertical Force [N]/1

== system spring_mass_model_01/Control/Behavior Control/Lateral PID Control/Lateral Hip PID ==
  position_error : Inport
  velocity_error : Inport  Port=2
  Discrete-Time Integrator : DiscreteIntegrator  IntegratorMethod=Integration: Trapezoidal  SampleTime=sample_time  LimitOutput=on  UpperSaturationLimit=i_limit_lateral  LowerSaturationLimit=-i_limit_lateral  ICPrevOutput=DiscIntNeverNeededParam  ICPrevScaledInput=DiscIntNeverNeededParam
  Sum : Sum  Inputs=+++
  kd_lateral : Gain  Description=xPCTag(1)=kd_lateral;  Gain=kd_lateral
  ki_lateral : Gain  Description=xPCTag(1)=ki_lateral;  Gain=ki_lateral
  kp_lateral : Gain  Description=xPCTag(1)=kp_lateral;  Gain=kp_lateral
  out : Outport
  wires:
  velocity_error/1 -> kd_lateral/1
  Discrete-Time Integrator/1 -> Sum/3
  ki_lateral/1 -> Discrete-Time Integrator/1
  kp_lateral/1 -> Sum/2
  position_error/1 -> ki_lateral/1, kp_lateral/1
  Sum/1 -> out/1
  kd_lateral/1 -> Sum/1

== system spring_mass_model_01/Control/Behavior Control/Lateral PID Control/spherical_correction_angle ==
  q_cmu : Inport
  Selector : Selector  InputPortWidth=13  Indices=[11]
  Sum1 : Sum  Inputs=|+-
  Terminator2 : Terminator
  boom_mount_angle : Constant  Value=boom_mount_angle
  lateral_correction : Gain  Gain=180/pi
  lateral_correction [rad] : Outport
  wires:
  Sum1/1 -> lateral_correction/1, lateral_correction [rad]/1
  Selector/1 -> Sum1/1  "qBoomRoll"
  q_cmu/1 -> Selector/1
  boom_mount_angle/1 -> Sum1/2
  lateral_correction/1 -> Terminator2/1

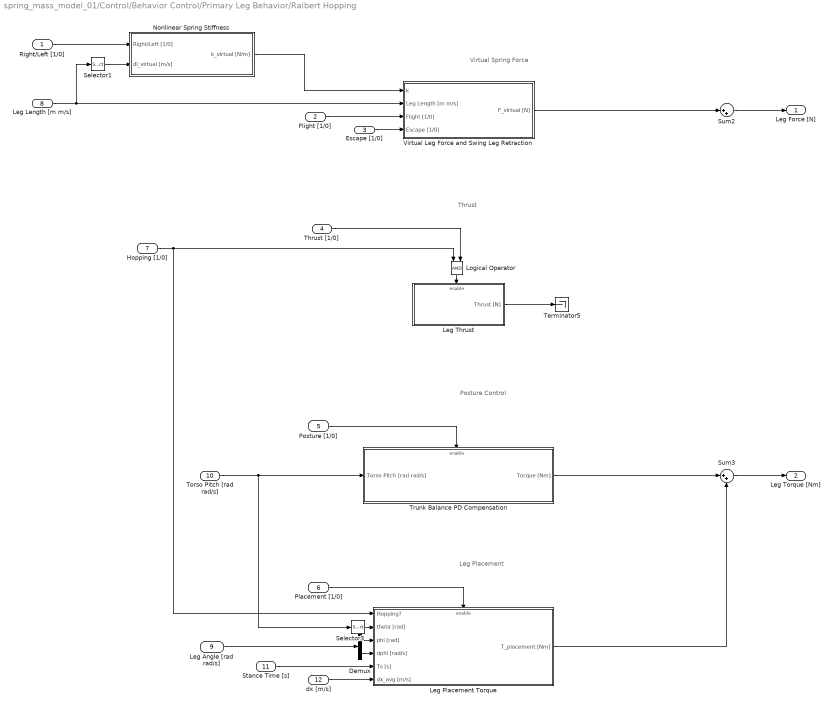
== system spring_mass_model_01/Control/Behavior Control/Primary Leg Behavior/Raibert Hopping ==
  note: Virtual Spring Force
  note: Thrust
  note: Posture Control
  note: Leg Placement
  Right/Left [1/0] : Inport
  Flight [1/0] : Inport  Port=2
  Escape [1/0] : Inport  Port=3
  Thrust [1/0] : Inport  Port=4
  Posture [1/0] : Inport  Port=5
  Placement [1/0] : Inport  Port=6
  Hopping [1/0] : Inport  Port=7
  Leg Length [m m/s] : Inport  Port=8
  Leg Angle [rad rad/s] : Inport  Port=9
  Torso Pitch [rad rad/s] : Inport  Port=10
  Stance Time [s] : Inport  Port=11
  dx [m/s] : Inport  Port=12
  Demux : Demux  Outputs=2
  Leg Placement Torque : Subsystem
  Leg Thrust : Subsystem
  Logical Operator : Logic  IconShape=distinctive  AllPortsSameDT=off  OutDataTypeStr=boolean
  Nonlinear Spring Stiffness : Subsystem
  Selector1 : Selector  InputPortWidth=2  Indices=[2]
  Selector3 : Selector  InputPortWidth=2  Indices=[1]
  Sum2 : Sum  Inputs=|++
  Sum3 : Sum  Inputs=|++
  Terminator5 : Terminator
  Trunk Balance PD Compensation : Subsystem
  Virtual Leg Force and Swing Leg Retraction : Subsystem
  Leg Force [N] : Outport
  Leg Torque [Nm] : Outport  Port=2
  wires:
  Sum2/1 -> Leg Force [N]/1
  Virtual Leg Force and Swing Leg Retraction/1(F_virtual [N]) -> Sum2/1
  Sum3/1 -> Leg Torque [Nm]/1
  Logical Operator/1 -> Leg Thrust/Enable
  Trunk Balance PD Compensation/1(Torque [Nm]) -> Sum3/1
  Leg Placement Torque/1(T_placement [Nm]) -> Sum3/2
  Stance Time [s]/1 -> Leg Placement Torque/5(Ts [s])
  dx [m/s]/1 -> Leg Placement Torque/6(dx_avg [m/s])
  Escape [1/0]/1 -> Virtual Leg Force and Swing Leg Retraction/4(Escape [1/0])
  Thrust [1/0]/1 -> Logical Operator/2
  Leg Length [m m/s]/1 -> Selector1/1, Virtual Leg Force and Swing Leg Retraction/2(Leg Length [m m/s])
  Posture [1/0]/1 -> Trunk Balance PD Compensation/Enable
  Leg Angle [rad rad/s]/1 -> Demux/1
  Torso Pitch [rad rad/s]/1 -> Trunk Balance PD Compensation/1(Torso Pitch [rad rad/s]), Selector3/1
  Selector3/1 -> Leg Placement Torque/2(theta [rad])
  Placement [1/0]/1 -> Leg Placement Torque/Enable
  Flight [1/0]/1 -> Virtual Leg Force and Swing Leg Retraction/3(Flight [1/0])
  Hopping [1/0]/1 -> Logical Operator/1, Leg Placement Torque/1(Hopping?)
  Demux/2 -> Leg Placement Torque/4(dphi [rad/s])
  Demux/1 -> Leg Placement Torque/3(phi [rad])
  Selector1/1 -> Nonlinear Spring Stiffness/2(dl_virtual [m/s])
  Nonlinear Spring Stiffness/1(k_virtual [N/m]) -> Virtual Leg Force and Swing Leg Retraction/1(k)
  Leg Thrust/1(Thrust [N]) -> Terminator5/1
  Right/Left [1/0]/1 -> Nonlinear Spring Stiffness/1(Right/Left [1/0])

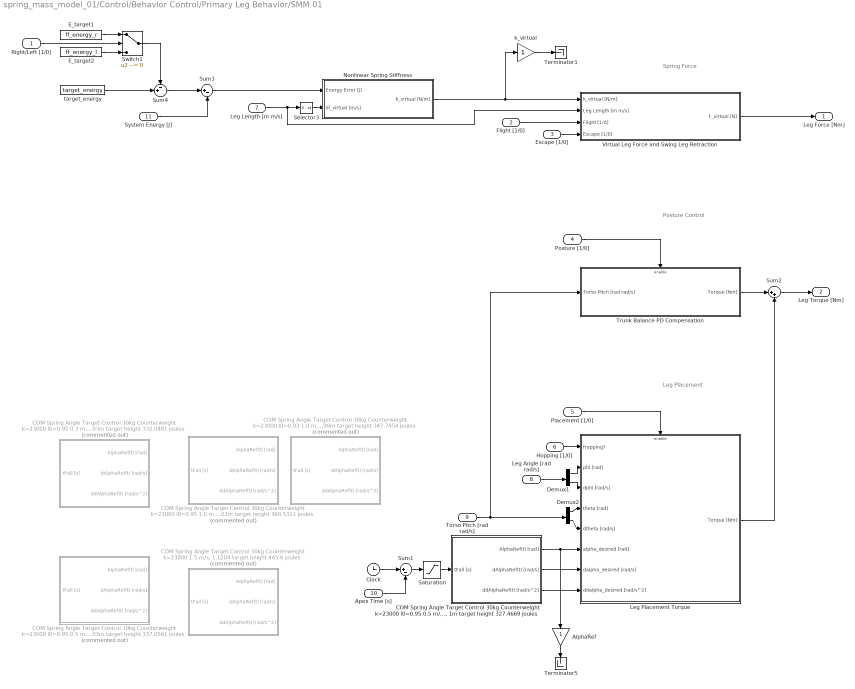
== system spring_mass_model_01/Control/Behavior Control/Primary Leg Behavior/SMM 01 ==
  note: Posture Control
  note: Leg Placement
  note: Spring Force
  Right/Left [1/0] : Inport
  Flight [1/0] : Inport  Port=2
  Escape [1/0] : Inport  Port=3
  Posture [1/0] : Inport  Port=4
  Placement [1/0] : Inport  Port=5
  Hopping [1/0] : Inport  Port=6
  Leg Length [m m/s] : Inport  Port=7
  Leg Angle [rad rad/s] : Inport  Port=8
  Torso Pitch [rad rad/s] : Inport  Port=9
  Apex Time [s] : Inport  Port=10
  System Energy [J] : Inport  Port=11
  AlphaRef : Gain
  "COM Spring Angle Target Control 30kg Counterweight k=23000 1.5 m/s, 1.1204 target height 445.6 joules" : Subsystem  Commented=on
  "COM Spring Angle Target Control 30kg Counterweight k=23000 l0=0.93 1.0 m/s, 0.99m target height 347.7454 joules" : Subsystem  Commented=on
  "COM Spring Angle Target Control 30kg Counterweight k=23000 l0=0.95 0.3 m/s, 1.03m target height 332.0481 joules" : Subsystem  Commented=on
  "COM Spring Angle Target Control 30kg Counterweight k=23000 l0=0.95 0.5 m/s, 1.03m target height 337.0561 joules" : Subsystem  Commented=on
  "COM Spring Angle Target Control 30kg Counterweight k=23000 l0=0.95 0.5 m/s, 1m target height 327.4669 joules" : Subsystem
  "COM Spring Angle Target Control 30kg Counterweight k=23000 l0=0.95 1.0 m/s, 1.03m target height 360.5311 joules" : Subsystem  Commented=on
  Clock : Clock
  Demux1 : Demux  Outputs=2
  Demux2 : Demux  Outputs=2
  E_target1 : Constant  Value=ff_energy_r
  E_target2 : Constant  Value=ff_energy_l
  Leg Placement Torque : Subsystem
  Nonlinear Spring Stiffness : Subsystem
  Saturation : Saturate  UpperLimit=3  LowerLimit=0
      settings: AttributesFormatString=|
      | Hi: %<UpperLimit>
      | Lo: %<LowerLimit>
  Selector3 : Selector  InputPortWidth=2  Indices=[2]
  Sum1 : Sum  Inputs=|+-
  Sum2 : Sum  Inputs=|++
  Sum3 : Sum  Inputs=|+-
  Sum4 : Sum  Inputs=-+|
  Switch1 : Switch  Criteria=u2 ~= 0
  Terminator1 : Terminator
  Terminator5 : Terminator
  Trunk Balance PD Compensation : Subsystem
  Virtual Leg Force and Swing Leg Retraction : Subsystem
  k_virtual : Gain
  target_energy : Constant  Value=target_energy
  Leg Force [Nm] : Outport
  Leg Torque [Nm] : Outport  Port=2
  wires:
  Selector3/1 -> Nonlinear Spring Stiffness/2(dl_virtual [m/s])
  Apex Time [s]/1 -> Sum1/2
  Sum1/1 -> Saturation/1
  Clock/1 -> Sum1/1
  "COM Spring Angle Target Control 30kg Counterweight k=23000 l0=0.95 0.5 m/s, 1m target height 327.4669 joules"/2(dAlphaRef(t) [rad/s]) -> Leg Placement Torque/7(dalpha_desired [rad/s])
  "COM Spring Angle Target Control 30kg Counterweight k=23000 l0=0.95 0.5 m/s, 1m target height 327.4669 joules"/3(ddAlphaRef(t) [rad/s^2]) -> Leg Placement Torque/8(ddalpha_desired [rad/s^2])
  Torso Pitch [rad rad/s]/1 -> Trunk Balance PD Compensation/1(Torso Pitch [rad rad/s]), Demux2/1
  "COM Spring Angle Target Control 30kg Counterweight k=23000 l0=0.95 0.5 m/s, 1m target height 327.4669 joules"/1(AlphaRef(t) [rad]) -> AlphaRef/1, Leg Placement Torque/6(alpha_desired [rad])
  AlphaRef/1 -> Terminator5/1
  Saturation/1 -> "COM Spring Angle Target Control 30kg Counterweight k=23000 l0=0.95 0.5 m/s, 1m target height 327.4669 joules"/1(tFall [s])
  Sum3/1 -> Nonlinear Spring Stiffness/1(Energy Error [J])
  Hopping [1/0]/1 -> Leg Placement Torque/1(Hopping?)
  Leg Length [m m/s]/1 -> Virtual Leg Force and Swing Leg Retraction/2(Leg Length [m m/s]), Selector3/1
  Escape [1/0]/1 -> Virtual Leg Force and Swing Leg Retraction/4(Escape [1/0])
  Placement [1/0]/1 -> Leg Placement Torque/Enable
  Leg Angle [rad rad/s]/1 -> Demux1/1
  Flight [1/0]/1 -> Virtual Leg Force and Swing Leg Retraction/3(Flight [1/0])
  Demux1/1 -> Leg Placement Torque/2(phi [rad])
  Demux1/2 -> Leg Placement Torque/3(dphi [rad/s])
  Demux2/1 -> Leg Placement Torque/4(theta [rad])
  Demux2/2 -> Leg Placement Torque/5(dtheta [rad/s])
  Posture [1/0]/1 -> Trunk Balance PD Compensation/Enable
  Sum2/1 -> Leg Torque [Nm]/1
  Trunk Balance PD Compensation/1(Torque [Nm]) -> Sum2/1
  Leg Placement Torque/1(Torque [Nm]) -> Sum2/2
  Virtual Leg Force and Swing Leg Retraction/1(F_virtual [N]) -> Leg Force [Nm]/1
  Nonlinear Spring Stiffness/1(k_virtual [N/m]) -> k_virtual/1, Virtual Leg Force and Swing Leg Retraction/1(k_virtual [N/m])
  k_virtual/1 -> Terminator1/1
  Sum4/1 -> Sum3/1
  System Energy [J]/1 -> Sum3/2
  Switch1/1 -> Sum4/1
  E_target1/1 -> Switch1/1
  E_target2/1 -> Switch1/3
  target_energy/1 -> Sum4/2
  Right/Left [1/0]/1 -> Switch1/2

== system spring_mass_model_01/Control/Behavior Control/Primary Secondary Leg Swap/Toggle ==
  Trigger : TriggerPort  TriggerType=falling  PortDimensions=1
  Logical Operator : Logic  Operator=NOT  AllPortsSameDT=off  OutDataTypeStr=boolean
  Memory : Memory  X0=1  InheritSampleTime=on
  "[1/0]" : Outport  InitialOutput=[1]
  wires:
  Logical Operator/1 -> "[1/0]"/1, Memory/1
  Memory/1 -> Logical Operator/1

== system spring_mass_model_01/Control/Behavior Control/Secondary Leg Behavior/Leg Angle PD ==
  Desired Angle : Inport
  Desired Velocity : Inport  Port=2
  Leg Angle [rad rad/s] : Inport  Port=3
  Demux1 : Demux  Outputs=2
  Gain6 : Gain  Gain=kp_leg_angle
  Gain7 : Gain  Gain=kd_leg_angle
  Sum7 : Sum  Inputs=|+-
  Sum8 : Sum  Inputs=|+-
  Sum9 : Sum  Inputs=|++
  Commanded Leg Torque [Nm] : Outport
  wires:
  Gain6/1 -> Sum9/1
  Sum7/1 -> Gain6/1
  Demux1/1 -> Sum7/2
  Sum9/1 -> Commanded Leg Torque [Nm]/1
  Desired Velocity/1 -> Sum8/1
  Sum8/1 -> Gain7/1
  Desired Angle/1 -> Sum7/1
  Gain7/1 -> Sum9/2
  Demux1/2 -> Sum8/2
  Leg Angle [rad rad/s]/1 -> Demux1/1

== system spring_mass_model_01/Control/Behavior Control/Secondary Leg Behavior/Leg Length PD ==
  Desired Length : Inport
  Desired Velocity : Inport  Port=2
  Leg Length [m m/s] : Inport  Port=3
  Demux1 : Demux  Outputs=2
  Sum7 : Sum  Inputs=|+-
  Sum8 : Sum  Inputs=|+-
  Sum9 : Sum
  kd_leg_length_secondary : Gain  Gain=kd_leg_length_secondary
  kp_leg_length_secondary : Gain  Gain=kp_leg_length_secondary
  Commanded Force [N] : Outport
  wires:
  Leg Length [m m/s]/1 -> Demux1/1
  Demux1/2 -> Sum8/2  "l_dot_measured"
  kd_leg_length_secondary/1 -> Sum9/2
  Desired Length/1 -> Sum7/1
  Sum8/1 -> kd_leg_length_secondary/1
  Desired Velocity/1 -> Sum8/1
  Sum9/1 -> Commanded Force [N]/1
  Demux1/1 -> Sum7/2  "l_measured"
  Sum7/1 -> kp_leg_length_secondary/1
  kp_leg_length_secondary/1 -> Sum9/1

== system spring_mass_model_01/Control/Behavior Control/Velocity Estimation/Recursive Moving Average ==
  Velocity [m/s] : Inport
  Delay : Delay  DelayLength=velocity_avg_samples  InitialCondition=0  UseCircularBuffer=on  SampleTime=sample_time
  Gain : Gain  Gain=1/velocity_avg_samples
  Sum : Sum  Inputs=-++
  Unit Delay : UnitDelay  SampleTime=sample_time
  Average Velocity [m/s] : Outport
  wires:
  Velocity [m/s]/1 -> Delay/1, Sum/2
  Sum/1 -> Unit Delay/1, Gain/1
  Delay/1 -> Sum/1
  Gain/1 -> Average Velocity [m/s]/1
  Unit Delay/1 -> Sum/3

== system spring_mass_model_01/Control/Behavior Control/Velocity Estimation/Signal During Escape ==
  signal : Inport
  time : Inport  Port=2
  Enable : EnablePort
  Trigger : TriggerPort  PortDimensions=1
  signal at escape : Outport
  time at escape : Outport  Port=2
  wires:
  signal/1 -> signal at escape/1
  time/1 -> time at escape/1

== system spring_mass_model_01/Control/Behavior Control/Velocity Estimation/Takeoff ==
  contact : Inport
  Compare To Constant : simulink/Logic and Bit Operations/Compare To Constant  relop=<=  const=TO_threshold  OutDataTypeStr=boolean
  Compare To Constant1 : simulink/Logic and Bit Operations/Compare To Constant  relop=>  const=TO_threshold  OutDataTypeStr=boolean
  Logical Operator : Logic  AllPortsSameDT=off  OutDataTypeStr=boolean
  Unit Delay1 : UnitDelay  SampleTime=sample_time
  takeoff : Outport
  wires:
  Compare To Constant1/1 -> Logical Operator/1
  Compare To Constant/1 -> Logical Operator/2
  contact/1 -> Compare To Constant/1, Unit Delay1/1
  Logical Operator/1 -> takeoff/1
  Unit Delay1/1 -> Compare To Constant1/1

== system spring_mass_model_01/Control/Behavior Control/Velocity Estimation/Takeoff Velocity ==
  Leg Length [m m/s] : Inport
  Leg Angle [rad rad/s] : Inport  Port=2
  Torso Pitch [rad rad/s] : Inport  Port=3
  Enable : EnablePort
  Demux2 : Demux  Outputs=2
  Demux3 : Demux  Outputs=2
  Demux4 : Demux  Outputs=2
  vertical_velocity : MATLAB Function  TreatAsAtomicUnit=on
  y_TO [m] : Outport  InitialOutput=[initial_com_height]
  dx_TO [m/s] : Outport  Port=2  InitialOutput=[initial_dx]
  dy_TO [m/s] : Outport  Port=3  InitialOutput=[0]
  wires:
  Demux2/1 -> vertical_velocity/1(l)
  Leg Length [m m/s]/1 -> Demux2/1
  Demux4/1 -> vertical_velocity/5(qPitch)
  Torso Pitch [rad rad/s]/1 -> Demux4/1
  Demux3/2 -> vertical_velocity/4(dphi)
  Demux3/1 -> vertical_velocity/3(phi)
  Leg Angle [rad rad/s]/1 -> Demux3/1
  Demux4/2 -> vertical_velocity/6(dqPitch)
  Demux2/2 -> vertical_velocity/2(dl)
  vertical_velocity/1(y) -> y_TO [m]/1
  vertical_velocity/2(dx) -> dx_TO [m/s]/1
  vertical_velocity/3(dy) -> dy_TO [m/s]/1
